simulink model "Ecocar_Challenge_Controls_Oct6EXPOchanges"  (R2015b)
settings: Solver=ode3  SolverMode=SingleTasking  StartTime=0.0  StopTime=10.0  RelTol=1e-3
libraries: arduinolib x4, simulink x1
settings Model: ExtModeTrigDuration=2  Creator=jessicatrac  LastModifiedBy=jessicatrac
settings DataIOCC: SaveFormat=Array
settings OptimizationCC: OptimizeModelRefInitCode=on  LifeSpan=1  MaxStackSize=64
settings DebuggingCC: UnderspecifiedInitializationDetection=Classic  MergeDetectMultiDrivingBlocksExec=none
settings HardwareCC: ProdBitPerInt=16  ProdBitPerPointer=16  ProdLargestAtomicFloat=None  ProdWordSize=8  ProdHWDeviceType=Atmel->AVR
settings RTWCC: SystemTargetFile=ert.tlc  TemplateMakefile=ert_default_tmf  Description=Embedded Coder  RTWVerbose=off  Toolchain=Arduino AVR v1.6.1  BuildConfiguration=Faster Runs
settings CodeAppCC: IgnoreCustomStorageClasses=off
settings ERTTargetCC: SupportContinuousTime=on  SupportVariableSizeSignals=on
settings ConfigComp: CovModelRefEnable=Off  CovSFcnEnable=off

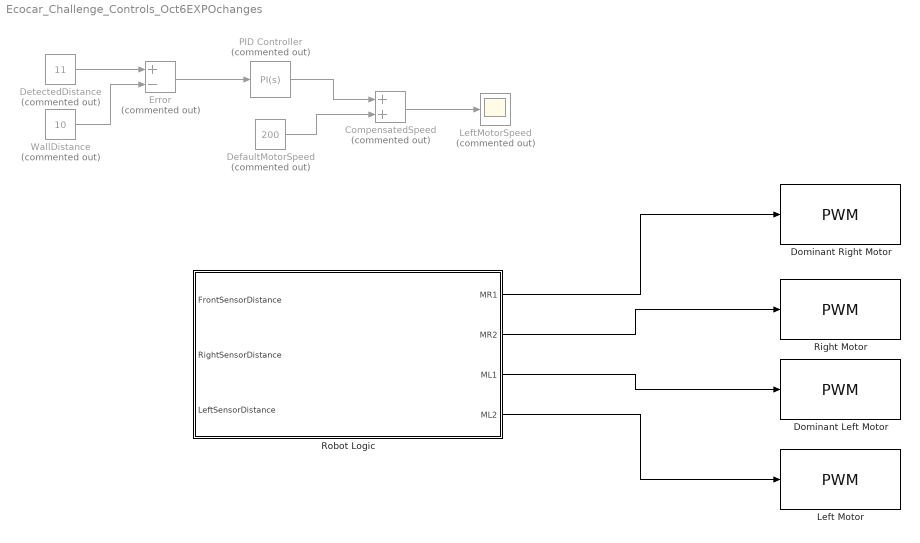
== system Ecocar_Challenge_Controls_Oct6EXPOchanges ==
  CompensatedSpeed : Sum  Commented=on
  DefaultMotorSpeed : Constant  Commented=on  Value=200
  "DetectedDistance " : Constant  Commented=on  Value=11
  Dominant Left Motor : arduinolib/PWM  pinNumber=5  blockPlatform=arduino
  Dominant Right Motor : arduinolib/PWM  pinNumber=9  blockPlatform=arduino
  Error : Sum  Commented=on  Inputs=+-
  Left Motor : arduinolib/PWM  pinNumber=3  blockPlatform=arduino
  LeftMotorSpeed : Scope  Commented=on
  PID Controller : simulink/Continuous/PID Controller  Commented=on  Controller=PI  TimeDomain=Continuous-time  SampleTime=-1  IntegratorMethod=Forward Euler  FilterMethod=Forward Euler  Form=Parallel  UseFilter=on  ControllerParametersSource=internal  P=1  I=1  D=0  N=100  InitialConditionSource=internal  InitialConditionForIntegrator=0  InitialConditionForFilter=0  ExternalReset=none  LimitOutput=off  UpperSaturationLimit=inf  LowerSaturationLimit=-inf  LinearizeAsGain=on  AntiWindupMode=none  Kb=1  TrackingMode=off  Kt=1  PParamMin=[]  PParamMax=[]  IParamMin=[]  IParamMax=[]  DParamMin=[]  DParamMax=[]  NParamMin=[]  NParamMax=[]  KbParamMin=[]  KbParamMax=[]  KtParamMin=[]  KtParamMax=[]  POutMin=[]  POutMax=[]  IOutMin=[]  IOutMax=[]  DOutMin=[]  DOutMax=[]  NOutMin=[]  NOutMax=[]  KbOutMin=[]  KbOutMax=[]  KtOutMin=[]  KtOutMax=[]  IntegratorOutMin=[]  IntegratorOutMax=[]  FilterOutMin=[]  FilterOutMax=[]  SumOutMin=[]  SumOutMax=[]  SumI1OutMin=[]  SumI1OutMax=[]  SumI2OutMin=[]  SumI2OutMax=[]  SumI3OutMin=[]  SumI3OutMax=[]  SumDOutMin=[]  SumDOutMax=[]  SaturationOutMin=[]  SaturationOutMax=[]  IntegratorContinuousStateAttributes=''  IntegratorStateMustResolveToSignalObject=off  IntegratorRTWStateStorageClass=Auto  FilterContinuousStateAttributes=''  FilterStateMustResolveToSignalObject=off  FilterRTWStateStorageClass=Auto  DifferentiatorICPrevScaledInput=0  DifferentiatorOutMin=[]  DifferentiatorOutMax=[]
  Right Motor : arduinolib/PWM  pinNumber=10  blockPlatform=arduino
  Robot Logic : Stateflow chart  TreatAsAtomicUnit=on
  WallDistance : Constant  Commented=on  Value=10
  wires:
  WallDistance/1 -> Error/2
  Error/1 -> PID Controller/1
  PID Controller/1 -> CompensatedSpeed/1
  DefaultMotorSpeed/1 -> CompensatedSpeed/2
  "DetectedDistance "/1 -> Error/1
  CompensatedSpeed/1 -> LeftMotorSpeed/1
  Robot Logic/1(MR1) -> Dominant Right Motor/1
  Robot Logic/2(MR2) -> Right Motor/1
  Robot Logic/3(ML1) -> Dominant Left Motor/1
  Robot Logic/4(ML2) -> Left Motor/1

== stateflow chart Ecocar_Challenge_Controls_Oct6EXPOchanges/Robot Logic ==
  state GoStraight
    entry: MR1 = 200; MR2 = 0;
    ML1 = 225; ML2 = 0;
  note: Motor speeds are varied to account for
      | uneven motors (calibrate for each robot)
  note: When front sensor detects clearance,
      | robot exits left turn mode and goes straight
  note: When front wall gets close, robot
      | will exit go straight mode and turn
  note: When front sensor detects clearance,
      | robot exits right turn mode and goes straight
  state TurnLeft
    entry: MR1 = 200; MR2 = 0;
    ML1 = 0; ML2 = 0;
  note: Junction is used so that when right/left are clear, robot will prefer a right turn.
      | If right wall is blocked, robot will turn left
  note: Turn off left motor and set right motor speed
      | to conduct left turn
  state TurnRight
    entry: MR1 = 0; MR2 = 0;
    ML1 = 225; ML2 = 0;
  note: Turn off right motor and set left motor speed
      | to conduct right turn
  note: 
  (default) -> GoStraight
  TurnLeft -> GoStraight : [FrontSensorDistance > 20]
  GoStraight -> (junction 59) : [FrontSensorDistance < 20]
  TurnRight -> GoStraight : [FrontSensorDistance > 20]
  (junction 59) -> TurnLeft [order 2] : [LeftSensorDistance > 20 && RightSensorDistance <= 20]
  (junction 59) -> TurnRight [order 1] : [RightSensorDistance > 20]
  data: FrontSensorDistance input; RightSensorDistance input; LeftSensorDistance input; MR1 output; MR2 output; ML1 output; ML2 output
